simulink model "newAttempt"  (R2024b)
settings: Solver=VariableStepAuto  StartTime=0.0  StopTime=2*N*ts  RelTol=1e-3
values from neighbouring files (symbols this model uses):
  B1 = 4    [TestWrapper.m]
  fin = 300/N*fs    (= 1373291.01562)    [TestWrapper.m]
  FSR = 2.4    [TestWrapper.m]
  G1 = 2^(B1-1)    (= 8)    [TestWrapper.m]
  magnitude = 1.2    [TestWrapper.m]
  ts = 1/fs    (= 3.33333333333e-09)    [TestWrapper.m]
  Vt_offset_en = false    [TestWrapper.m]
  Vt_var = 0.0    (= 0)    [TestWrapper.m]
settings Model: Creator=bbassett6  LastModifiedBy=bbassett6

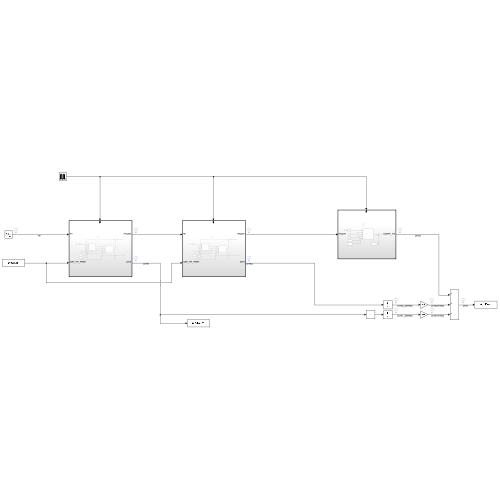
[thumbnail: Simulink's stored preview of the top-level diagram]
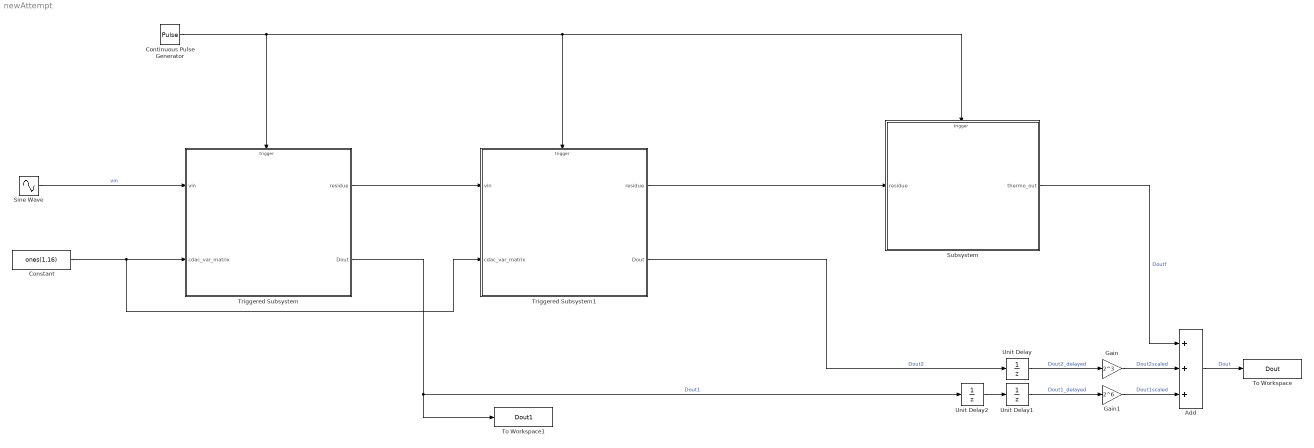
== system newAttempt ==
  Add : Sum  Inputs=+++
  Constant : Constant  Value=ones(1,16)  VectorParams1D=off
  Continuous Pulse Generator : DiscretePulseGenerator  PulseType=Time based  Period=ts  PulseWidth=50
  Gain : Gain  Gain=2^3
  Gain1 : Gain  Gain=2^6
  Sine Wave : Sin  Amplitude=magnitude  Bias=1e-5  Frequency=2*pi*fin  SampleTime=0
  Subsystem : Subsystem
  To Workspace : ToWorkspace  VariableName=Dout  SampleTime=ts
  To Workspace1 : ToWorkspace  VariableName=Dout1  SampleTime=ts
  Triggered Subsystem : Subsystem  TreatAsAtomicUnit=on
  Triggered Subsystem1 : Subsystem  TreatAsAtomicUnit=on
  Unit Delay : UnitDelay  SampleTime=ts/2  HasFrameUpgradeWarning=on
  Unit Delay1 : UnitDelay  SampleTime=ts/2  HasFrameUpgradeWarning=on
  Unit Delay2 : UnitDelay  SampleTime=ts/2  HasFrameUpgradeWarning=on
  wires:
  Sine Wave/1 -> Triggered Subsystem/1(vin)  "vin"
  Triggered Subsystem/2(Dout) -> To Workspace1/1, Unit Delay2/1  "Dout1"
  Continuous Pulse Generator/1 -> Triggered Subsystem1/Trigger, Subsystem/Trigger, Triggered Subsystem/Trigger
  Subsystem/1(thermo_out) -> Add/1  "Doutf"
  Gain/1 -> Add/2  "Dout2scaled"
  Add/1 -> To Workspace/1  "Dout"
  Unit Delay/1 -> Gain/1  "Dout2_delayed"
  Constant/1 -> Triggered Subsystem1/2(cdac_var_matrix), Triggered Subsystem/2(cdac_var_matrix)
  Triggered Subsystem/1(residue) -> Triggered Subsystem1/1(vin)
  Triggered Subsystem1/1(residue) -> Subsystem/1(residue)
  Gain1/1 -> Add/3  "Dout1scaled"
  Unit Delay1/1 -> Gain1/1  "Dout1_delayed"
  Unit Delay2/1 -> Unit Delay1/1
  Triggered Subsystem1/2(Dout) -> Unit Delay/1  "Dout2"

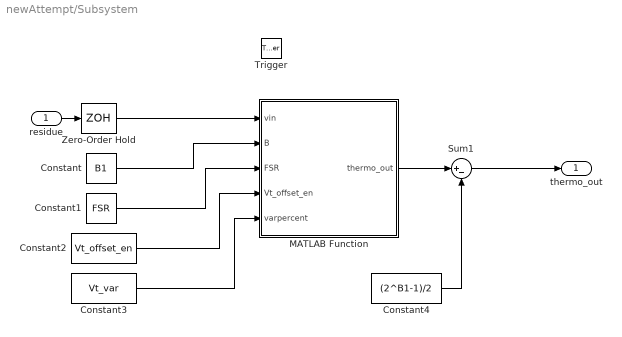
== system newAttempt/Subsystem ==
  residue : Inport
  Trigger : TriggerPort  VariantControl=(inherit)  PortDimensions=1
  Constant : Constant  Value=B1
  Constant1 : Constant  Value=FSR
  Constant2 : Constant  Value=Vt_offset_en
  Constant3 : Constant  Value=Vt_var
  Constant4 : Constant  Value=(2^B1-1)/2
  MATLAB Function : MATLAB Function  TreatAsAtomicUnit=on
  Sum1 : Sum  Inputs=|+-
  Zero-Order Hold : ZeroOrderHold  SampleTime=-1
  thermo_out : Outport
  wires:
  residue/1 -> Zero-Order Hold/1
  Constant3/1 -> MATLAB Function/5(varpercent)
  Constant1/1 -> MATLAB Function/3(FSR)
  Constant2/1 -> MATLAB Function/4(Vt_offset_en)
  Zero-Order Hold/1 -> MATLAB Function/1(vin)
  Constant/1 -> MATLAB Function/2(B)
  Constant4/1 -> Sum1/2
  MATLAB Function/1(thermo_out) -> Sum1/1
  Sum1/1 -> thermo_out/1

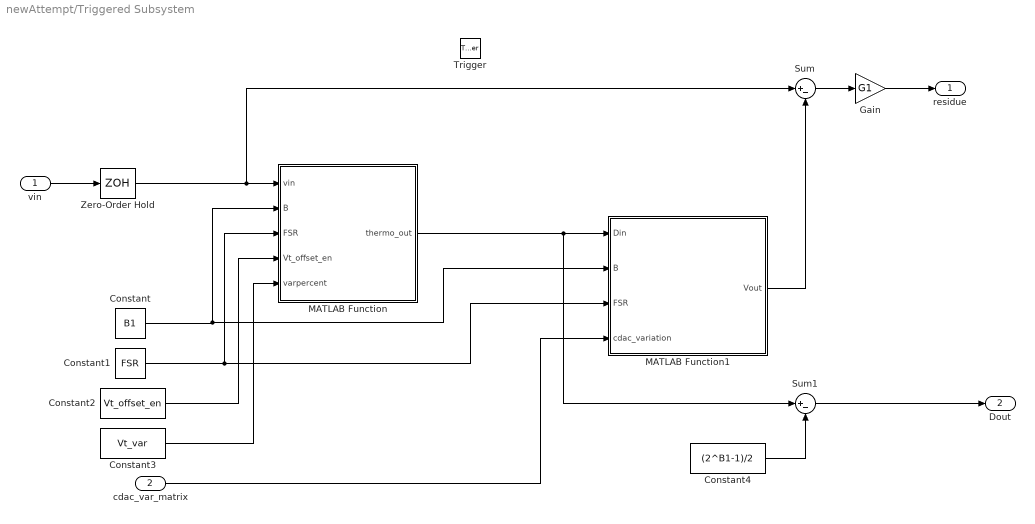
== system newAttempt/Triggered Subsystem ==
  vin : Inport
  cdac_var_matrix : Inport  Port=2
  Trigger : TriggerPort  VariantControl=(inherit)
  Constant : Constant  Value=B1
  Constant1 : Constant  Value=FSR
  Constant2 : Constant  Value=Vt_offset_en
  Constant3 : Constant  Value=Vt_var
  Constant4 : Constant  Value=(2^B1-1)/2
  Gain : Gain  Gain=G1
  MATLAB Function : MATLAB Function  TreatAsAtomicUnit=on
  MATLAB Function1 : MATLAB Function  TreatAsAtomicUnit=on
  Sum : Sum  Inputs=|+-
  Sum1 : Sum  Inputs=|+-
  Zero-Order Hold : ZeroOrderHold  SampleTime=-1
  residue : Outport
  Dout : Outport  Port=2
  wires:
  MATLAB Function/1(thermo_out) -> Sum1/1, MATLAB Function1/1(Din)
  vin/1 -> Zero-Order Hold/1
  MATLAB Function1/1(Vout) -> Sum/2
  Sum/1 -> Gain/1
  Gain/1 -> residue/1
  Constant/1 -> MATLAB Function1/2(B), MATLAB Function/2(B)
  Constant1/1 -> MATLAB Function1/3(FSR), MATLAB Function/3(FSR)
  Zero-Order Hold/1 -> Sum/1, MATLAB Function/1(vin)
  Constant2/1 -> MATLAB Function/4(Vt_offset_en)
  Constant3/1 -> MATLAB Function/5(varpercent)
  cdac_var_matrix/1 -> MATLAB Function1/4(cdac_variation)
  Sum1/1 -> Dout/1
  Constant4/1 -> Sum1/2

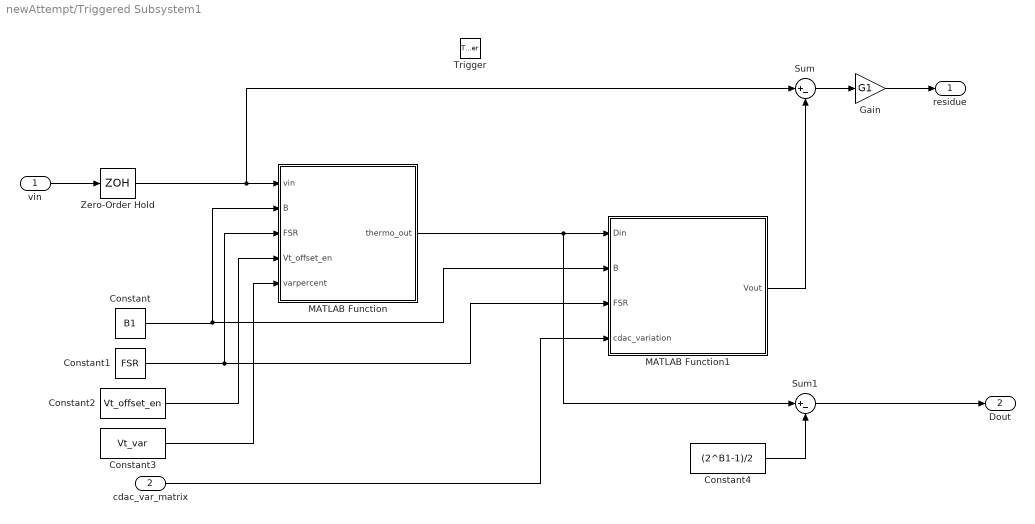
== system newAttempt/Triggered Subsystem1 ==
  vin : Inport
  cdac_var_matrix : Inport  Port=2
  Trigger : TriggerPort  TriggerType=falling  VariantControl=(inherit)
  Constant : Constant  Value=B1
  Constant1 : Constant  Value=FSR
  Constant2 : Constant  Value=Vt_offset_en
  Constant3 : Constant  Value=Vt_var
  Constant4 : Constant  Value=(2^B1-1)/2
  Gain : Gain  Gain=G1
  MATLAB Function : MATLAB Function  TreatAsAtomicUnit=on
  MATLAB Function1 : MATLAB Function  TreatAsAtomicUnit=on
  Sum : Sum  Inputs=|+-
  Sum1 : Sum  Inputs=|+-
  Zero-Order Hold : ZeroOrderHold  SampleTime=-1
  residue : Outport
  Dout : Outport  Port=2
  wires:
  MATLAB Function/1(thermo_out) -> Sum1/1, MATLAB Function1/1(Din)
  vin/1 -> Zero-Order Hold/1
  MATLAB Function1/1(Vout) -> Sum/2
  Sum/1 -> Gain/1
  Gain/1 -> residue/1
  Constant/1 -> MATLAB Function1/2(B), MATLAB Function/2(B)
  Constant1/1 -> MATLAB Function1/3(FSR), MATLAB Function/3(FSR)
  Zero-Order Hold/1 -> Sum/1, MATLAB Function/1(vin)
  Constant2/1 -> MATLAB Function/4(Vt_offset_en)
  Constant3/1 -> MATLAB Function/5(varpercent)
  cdac_var_matrix/1 -> MATLAB Function1/4(cdac_variation)
  Sum1/1 -> Dout/1
  Constant4/1 -> Sum1/2

== matlab function newAttempt/Triggered Subsystem/MATLAB Function1 ==
  data: Din input; Vout output size=1; B input; FSR input; cdac_variation input
function Vout = Cdac(Din, B, FSR, cdac_variation)

% LSB = FSR/2^B;

y = [1 1 2 4 8 16 32 64 128 256 512 1024 2048 4096];

Cdac_array = y(1:B+1).*cdac_variation(1:B+1);
Cdac_array = flip(Cdac_array);

Dout = dec2bin(Din*2,B+1);
Dout_num = ones(length(Dout),1);

for n=1:length(Dout)
    if abs(str2double(Dout(n)))==1
        Dout_num(n) = abs(str2double(Dout(n)));
    else
        Dout_num(n) = -1;
    end
end
Dout_num(B+1) = 0;
Dout_num;
VOUT = Cdac_array*Dout_num/(sum(Cdac_array));
Vout = sum(VOUT*FSR/2);
% VOUT = cast(Vout, "double");
% Cdac.outputs(1).DataType = 'double';

end

== matlab function newAttempt/Triggered Subsystem/MATLAB Function ==
  data: vin input; thermo_out output; B input; FSR input; Vt_offset_en input; varpercent input
function thermo_out = flash_qtz(vin, B, FSR, Vt_offset_en, varpercent)

LSB = FSR/2^B;

variation = rand(1,2^B-1);
variation = variation-0.5;
variation = variation.*varpercent;
vt_variation = variation+1;

Vtrans = -FSR/2+LSB:LSB:FSR/2-LSB;

if Vt_offset_en
    Vtrans = Vtrans + 0.01*Vtrans.^2 + 0.01*Vtrans.^3;
end

Vtrans = Vtrans.*vt_variation;

thermo_out = sum(vin>Vtrans);

end

== matlab function newAttempt/Subsystem/MATLAB Function ==
  data: vin input; thermo_out output; B input; FSR input; Vt_offset_en input; varpercent input
function thermo_out = flash_qtz(vin, B, FSR, Vt_offset_en, varpercent)

LSB = FSR/2^B;

variation = rand(1,2^B-1);
variation = variation-0.5;
variation = variation.*varpercent;
vt_variation = variation+1;

Vtrans = -FSR/2+LSB:LSB:FSR/2-LSB;

if Vt_offset_en
    Vtrans = Vtrans + 0.01*Vtrans.^2 + 0.01*Vtrans.^3;
end

Vtrans = Vtrans.*vt_variation;

thermo_out = sum(vin>Vtrans);

end

== matlab function newAttempt/Triggered Subsystem1/MATLAB Function ==
  data: vin input; thermo_out output; B input; FSR input; Vt_offset_en input; varpercent input
function thermo_out = flash_qtz(vin, B, FSR, Vt_offset_en, varpercent)

LSB = FSR/2^B;

variation = rand(1,2^B-1);
variation = variation-0.5;
variation = variation.*varpercent;
vt_variation = variation+1;

Vtrans = -FSR/2+LSB:LSB:FSR/2-LSB;

if Vt_offset_en
    Vtrans = Vtrans + 0.01*Vtrans.^2 + 0.01*Vtrans.^3;
end

Vtrans = Vtrans.*vt_variation;

thermo_out = sum(vin>Vtrans);

end

== matlab function newAttempt/Triggered Subsystem1/MATLAB Function1 ==
  data: Din input; Vout output size=1; B input; FSR input; cdac_variation input
function Vout = Cdac(Din, B, FSR, cdac_variation)

% LSB = FSR/2^B;

y = [1 1 2 4 8 16 32 64 128 256 512 1024 2048 4096];

Cdac_array = y(1:B+1).*cdac_variation(1:B+1);
Cdac_array = flip(Cdac_array);

Dout = dec2bin(Din*2,B+1);
Dout_num = ones(length(Dout),1);

for n=1:length(Dout)
    if abs(str2double(Dout(n)))==1
        Dout_num(n) = abs(str2double(Dout(n)));
    else
        Dout_num(n) = -1;
    end
end
Dout_num(B+1) = 0;
Dout_num;
VOUT = Cdac_array*Dout_num/(sum(Cdac_array));
Vout = sum(VOUT*FSR/2);
% VOUT = cast(Vout, "double");
% Cdac.outputs(1).DataType = 'double';

end
